simulink model "simple"  (R2013b)
settings: Solver=FixedStepDiscrete  StartTime=0.0  StopTime=inf  FixedStep=900  RelTol=1e-3
undefined symbols (not defined in the file or in its folder): OHare, USA_IL_Chicago
libraries: mlepLibrary x1, simulink x1
settings Model: ExtModeAutoUpdateStatusClock=off  Creator=mwetter  LastModifiedBy=wbernalh
settings DataIOCC: SignalLoggingSaveFormat=ModelDataLogs
settings OptimizationCC: ExpressionDepthLimit=2147483647  InitFltsAndDblsToZero=on  SimCompilerOptimization=off
settings DebuggingCC: SaveWithParameterizedLinksMsg=none  FcnCallInpInsideContextMsg=EnableAllAsWarning  FrameProcessingCompatibilityMsg=error  StateNameClashWarn=warning
settings SFSimCC: SimParseCustomCode=off
settings RTWCC: RTWCompilerOptimization=off
settings GRTTargetCC: TargetFcnLib=ansi_tfl_tmw.mat  TargetLangStandard=C89/C90 (ANSI)  CodeReplacementLibrary=None  CombineOutputUpdateFcns=off  CPPClassGenCompliant=on  GRTInterface=on

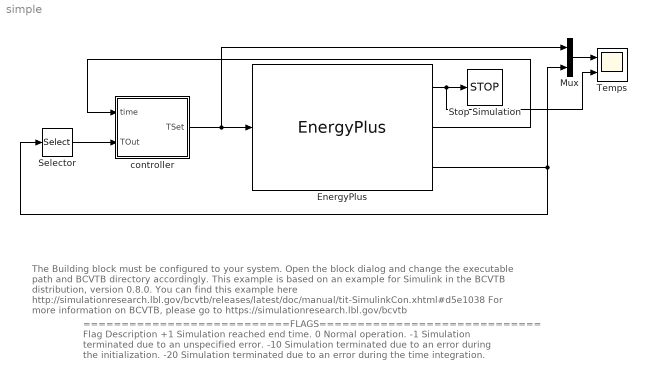
== system simple ==
  note: ===========================FLAGS=============================
      | Flag	Description
      | +1	Simulation reached end time.
      | 0	Normal operation.
      | -1	Simulation terminated due to an unspecified error.
      | -10	Simulation terminated due to an error during the initialization.
      | -20	Simulation terminated due to an error during the time integration.
  note: The Building block must be configured to your system.
      | Open the block dialog and change the executable path and BCVTB directory accordingly.
      |
      | This example is based on an example for Simulink in the BCVTB distribution, version 0.8.0.
      | You can find this example here http://simulationresearch.lbl.gov/bcvtb/releases/latest/doc/manual/tit-SimulinkCon.xhtml#d5e1038
      | For more information on BCVTB, please go to https://simulationresearch.lbl.gov/bcvtb
  EnergyPlus : mlepLibrary/EnergyPlus  rel_path=on  fname=SmOffPSZ  weather_profile=USA_IL_Chicago-OHare.Intl.AP.725300_TMY3  time_step=900  nout=2  timeout=10  mlep_defaults=on  port=0
  Mux : Mux  Inputs=2
  Selector : Selector  InputPortWidth=2  IndexOptions=Index vector (dialog)  Indices=[1]  OutputSizes=1
  Stop Simulation : Stop
  Temps : Scope  NumInputPorts=2
      settings: TimeRange=346500  YMin=0~-5  YMax=35~5
  controller : Subsystem
  wires:
  controller/1(TSet) -> EnergyPlus/1, Mux/1
  EnergyPlus/2 -> controller/1(time)
  EnergyPlus/1 -> Temps/2, Stop Simulation/1
  EnergyPlus/3 -> Mux/2, Selector/1
  Mux/1 -> Temps/1
  Selector/1 -> controller/2(TOut)

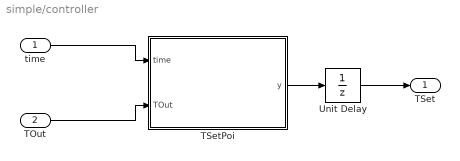
== system simple/controller ==
  time : Inport
  TOut : Inport  Port=2
  TSetPoi : Subsystem
  Unit Delay : UnitDelay  SampleTime=-1
  TSet : Outport
  wires:
  time/1 -> TSetPoi/1(time)
  TOut/1 -> TSetPoi/2(TOut)
  Unit Delay/1 -> TSet/1
  TSetPoi/1(y) -> Unit Delay/1

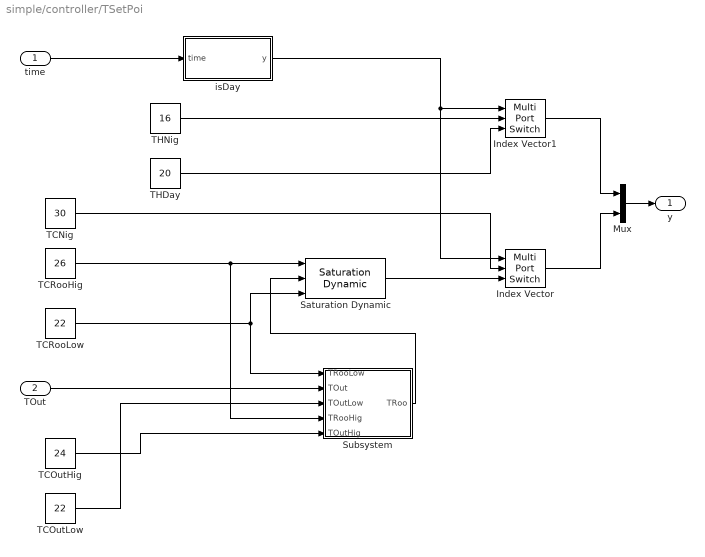
== system simple/controller/TSetPoi ==
  time : Inport
  TOut : Inport  Port=2
  Index Vector : MultiPortSwitch  DataPortOrder=Zero-based contiguous  Inputs=2  zeroidx=on
  Index Vector1 : MultiPortSwitch  DataPortOrder=Zero-based contiguous  Inputs=2  zeroidx=on
  Mux : Mux  Inputs=2
  Saturation Dynamic : simulink/Discontinuities/Saturation Dynamic  OutMin=[]  OutMax=[]  OutDataTypeStr=Inherit: Same as second input  OutDataType=sfix(16)  OutScaling=2^-10  DoSatur=off
  Subsystem : Subsystem
  TCNig : Constant  Value=30
  TCOutHig : Constant  Value=24
  TCOutLow : Constant  Value=22
  TCRooHig : Constant  Value=26
  TCRooLow : Constant  Value=22
  THDay : Constant  Value=20
  THNig : Constant  Value=16
  isDay : Subsystem
  y : Outport
  wires:
  TOut/1 -> Subsystem/2(TOut)
  TCOutLow/1 -> Subsystem/3(TOutLow)
  TCOutHig/1 -> Subsystem/5(TOutHig)
  TCRooHig/1 -> Saturation Dynamic/1, Subsystem/4(TRooHig)
  TCRooLow/1 -> Saturation Dynamic/3, Subsystem/1(TRooLow)
  time/1 -> isDay/1(time)
  isDay/1(y) -> Index Vector/1, Index Vector1/1
  TCNig/1 -> Index Vector/2
  Subsystem/1(TRoo) -> Saturation Dynamic/2
  Saturation Dynamic/1 -> Index Vector/3
  THNig/1 -> Index Vector1/2
  THDay/1 -> Index Vector1/3
  Index Vector1/1 -> Mux/1
  Index Vector/1 -> Mux/2
  Mux/1 -> y/1

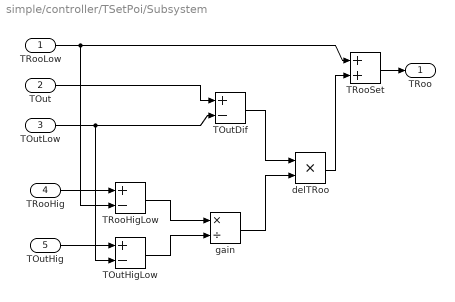
== system simple/controller/TSetPoi/Subsystem ==
  TRooLow : Inport
  TOut : Inport  Port=2
  TOutLow : Inport  Port=3
  TRooHig : Inport  Port=4
  TOutHig : Inport  Port=5
  TOutDif : Sum  Inputs=+-
  TOutHigLow : Sum  Inputs=+-
  TRooHigLow : Sum  Inputs=+-
  TRooSet : Sum
  delTRoo : Product  RndMeth=Zero
  gain : Product  Inputs=*/
  TRoo : Outport
  wires:
  TRooHigLow/1 -> gain/1
  TOutHigLow/1 -> gain/2
  TOutDif/1 -> delTRoo/1
  gain/1 -> delTRoo/2
  delTRoo/1 -> TRooSet/2
  TRooLow/1 -> TRooSet/1, TRooHigLow/2
  TOutLow/1 -> TOutDif/2, TOutHigLow/2
  TRooHig/1 -> TRooHigLow/1
  TOutHig/1 -> TOutHigLow/1
  TRooSet/1 -> TRoo/1
  TOut/1 -> TOutDif/1

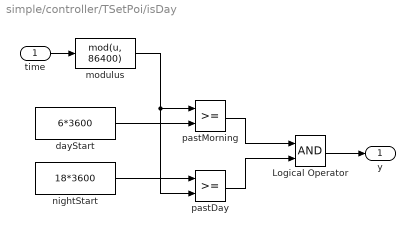
== system simple/controller/TSetPoi/isDay ==
  time : Inport
  Logical Operator : Logic  AllPortsSameDT=off  OutDataTypeStr=boolean
  dayStart : Constant  Value=6*3600
  modulus : MATLABFcn  MATLABFcn=mod(u, 86400)
  nightStart : Constant  Value=18*3600
  pastDay : RelationalOperator  OutDataTypeStr=boolean
  pastMorning : RelationalOperator  OutDataTypeStr=boolean
  y : Outport
  wires:
  time/1 -> modulus/1
  modulus/1 -> pastMorning/1, pastDay/2
  dayStart/1 -> pastMorning/2
  nightStart/1 -> pastDay/1
  pastMorning/1 -> Logical Operator/1
  pastDay/1 -> Logical Operator/2
  Logical Operator/1 -> y/1
